simulink subsystem "Actuator"  (R2023b)
settings: Solver=VariableStepAuto  StartTime=0.0  StopTime=10.0  RelTol=1e-3
values from neighbouring files (symbols this model uses):
  a = 0.002    [Diplomm.m]
  c = 490873    [Diplomm.m]
  F1 = 0.003    [Diplomm.m]
  F2 = 0.003    [Diplomm.m]
  G = 0.15    [Diplomm.m]
  G1 = 0.06    [Diplomm.m]
  G2 = 0.16    [Diplomm.m]
  i = 619    [Diplomm.m]
  Jd = 4.4e-6    (= 4.4e-06)    [Diplomm.m]
  Km = 0.077    [Diplomm.m]
  Kw = 0.091    [Diplomm.m]
  L = 1.05e-3    (= 0.00105)    [Diplomm.m]
  R = 1.8    [Diplomm.m]
settings Model: Creator=mrrom  LastModifiedBy=mrrom

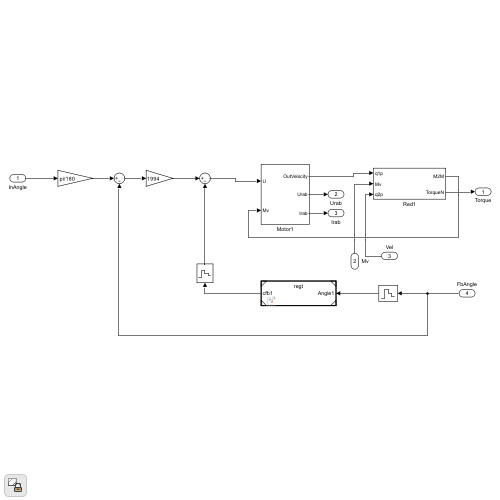
[thumbnail: Simulink's stored preview of the top-level diagram]
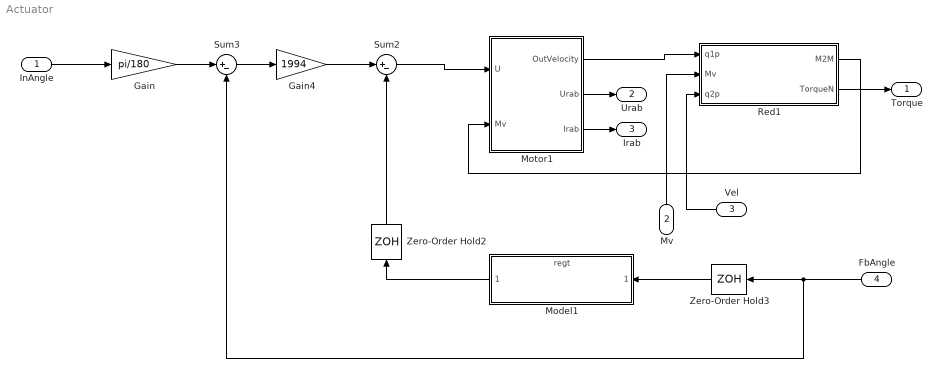
== system Actuator ==
  InAngle : Inport
  Mv : Inport  Port=2
  Vel : Inport  Port=3
  FbAngle : Inport  Port=4
  Gain : Gain  Gain=pi/180
  Gain4 : Gain  Gain=1994
  Model1 : ModelReference  ModelNameDialog=regt.slx  SimulationMode=Normal  ModelReferenceVersion=1.14  OutputSignalHandling=Zero-order hold
  Motor1 : Subsystem
  Red1 : Subsystem
  Sum2 : Sum  Inputs=|+-
  Sum3 : Sum  Inputs=|+-
  Zero-Order Hold2 : ZeroOrderHold  SampleTime=0.01
  Zero-Order Hold3 : ZeroOrderHold  SampleTime=0.01
  Torque : Outport
  Urab : Outport  Port=2
  Irab : Outport  Port=3
  wires:
  Gain4/1 -> Sum2/1
  Model1/1 -> Zero-Order Hold2/1
  Zero-Order Hold3/1 -> Model1/1
  Red1/1(M2M) -> Motor1/2(Mv)
  Motor1/1(OutVelocity) -> Red1/1(q1p)
  Zero-Order Hold2/1 -> Sum2/2
  Gain/1 -> Sum3/1
  InAngle/1 -> Gain/1
  Mv/1 -> Red1/2(Mv)
  Vel/1 -> Red1/3(q2p)
  Red1/2(TorqueN) -> Torque/1
  Sum3/1 -> Gain4/1
  FbAngle/1 -> Sum3/2, Zero-Order Hold3/1
  Sum2/1 -> Motor1/1(U)
  Motor1/2(Urab) -> Urab/1
  Motor1/3(Irab) -> Irab/1

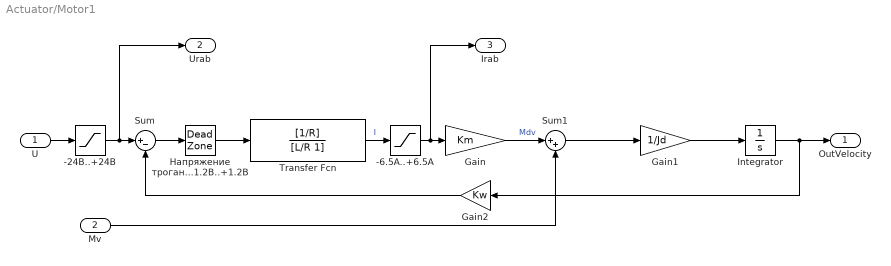
== system Actuator/Motor1 ==
  U : Inport
  Mv : Inport  Port=2
  -24В..+24В : Saturate  UpperLimit=24  LowerLimit=-24
  -6.5A..+6.5A : Saturate  UpperLimit=6.5  LowerLimit=-6.5
  Gain : Gain  Gain=Km
  Gain1 : Gain  Gain=1/Jd
  Gain2 : Gain  Gain=Kw
  Integrator : Integrator
  Sum : Sum  Inputs=|+-
  Sum1 : Sum  Inputs=|++
  Transfer Fcn : TransferFcn  Numerator=[1/R]  Denominator=[L/R 1]
  Напряжение трогания -1.2В..+1.2В : DeadZone  LowerValue=-1.2  UpperValue=1.2
  OutVelocity : Outport
  Urab : Outport  Port=2
  Irab : Outport  Port=3
  wires:
  Напряжение трогания -1.2В..+1.2В/1 -> Transfer Fcn/1
  Sum/1 -> Напряжение трогания -1.2В..+1.2В/1
  -6.5A..+6.5A/1 -> Gain/1, Irab/1
  -24В..+24В/1 -> Sum/1, Urab/1
  Sum1/1 -> Gain1/1
  Gain1/1 -> Integrator/1
  Integrator/1 -> Gain2/1, OutVelocity/1
  Mv/1 -> Sum1/2
  U/1 -> -24В..+24В/1
  Gain/1 -> Sum1/1  "Mdv"
  Gain2/1 -> Sum/2
  Transfer Fcn/1 -> -6.5A..+6.5A/1  "I"

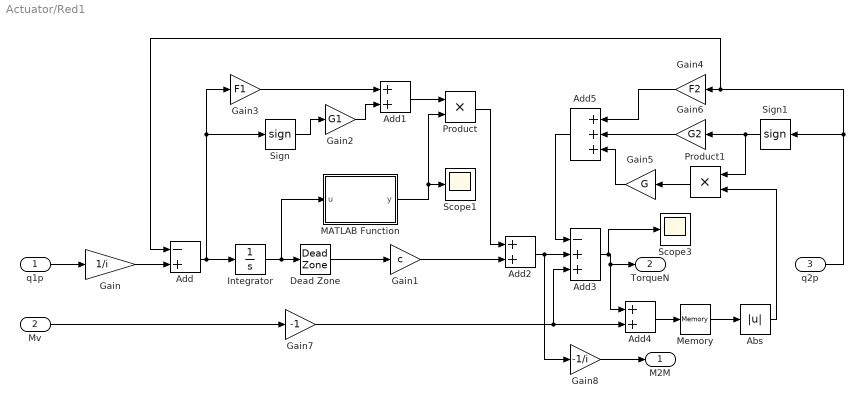
== system Actuator/Red1 ==
  q1p : Inport
  Mv : Inport  Port=2
  q2p : Inport  Port=3
  Abs : Abs  SaturateOnIntegerOverflow=off
  Add : Sum  Inputs=-+
  Add1 : Sum
  Add2 : Sum
  Add3 : Sum  Inputs=-++
  Add4 : Sum
  Add5 : Sum  Inputs=+++
  Dead Zone : DeadZone  LowerValue=-a  UpperValue=a
  Gain : Gain  Gain=1/i
  Gain1 : Gain  Gain=c
  Gain2 : Gain  Gain=G1
  Gain3 : Gain  Gain=F1
  Gain4 : Gain  Gain=F2
  Gain5 : Gain  Gain=G
  Gain6 : Gain  Gain=G2
  Gain7 : Gain  Gain=-1
  Gain8 : Gain  Gain=-1/i
  Integrator : Integrator
  MATLAB Function : MATLAB Function  TreatAsAtomicUnit=on
  Memory : Memory
  Product : Product
  Product1 : Product
  Scope1 : Scope
  Scope3 : Scope
  Sign : Signum  ZeroCross=off
  Sign1 : Signum  ZeroCross=off
  M2M : Outport
  TorqueN : Outport  Port=2
  wires:
  q2p/1 -> Sign1/1, Gain4/1, Add/1
  Memory/1 -> Abs/1
  MATLAB Function/1(y) -> Product/2, Scope1/1
  Gain7/1 -> Add3/3, Add4/2
  Add4/1 -> Memory/1
  Gain8/1 -> M2M/1
  Abs/1 -> Product1/2
  Sign1/1 -> Gain6/1, Product1/1
  Product1/1 -> Gain5/1
  Gain5/1 -> Add5/3
  Gain6/1 -> Add5/2
  Gain4/1 -> Add5/1
  Add5/1 -> Add3/1
  Add3/1 -> Add4/1, TorqueN/1, Scope3/1
  Mv/1 -> Gain7/1
  Add2/1 -> Gain8/1, Add3/2
  Gain1/1 -> Add2/2
  Product/1 -> Add2/1
  Add1/1 -> Product/1
  Gain3/1 -> Add1/1
  Gain2/1 -> Add1/2
  Sign/1 -> Gain2/1
  Dead Zone/1 -> Gain1/1
  Integrator/1 -> Dead Zone/1, MATLAB Function/1(u)
  Add/1 -> Sign/1, Gain3/1, Integrator/1
  Gain/1 -> Add/2
  q1p/1 -> Gain/1

== matlab function Actuator/Red1/MATLAB Function ==
  data: u input; y output
function y = fcn(u)
if abs(u) <= 0.002
    y = 0;
else
    y = 1;
end
